simulink model "derivative_filter_test"  (R2023a)
settings: Solver=FixedStepDiscrete  StartTime=0.0  StopTime=1  FixedStep=T_s  RelTol=1e-3
InitFcn:
  | filter_init
values from neighbouring files (symbols this model uses):
  beta_v = T_s/(T_s+tau_v)    (= 0.5)    [filter_init.m]
  N_e = 12    [filter_init.m]
  T_s = 0.001    [filter_init.m]
  tau_der = 0.01    [filter_init.m]
undefined symbols (not defined in the file or in its folder): den_filt, den_filt_be, den_filt_fe, num_filt, num_filt_be, num_filt_fe
settings Model: Creator=mfocchi  LastModifiedBy=mfocchi

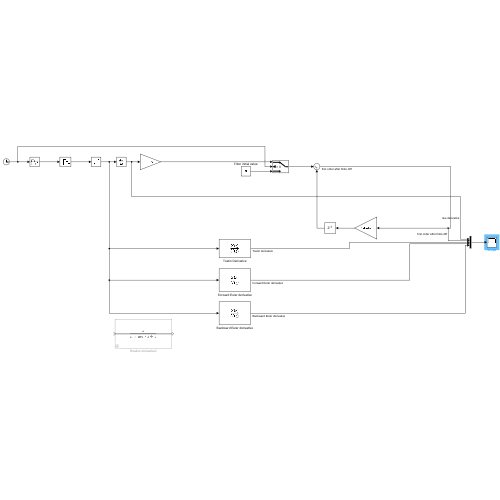
[thumbnail: Simulink's stored preview of the top-level diagram]
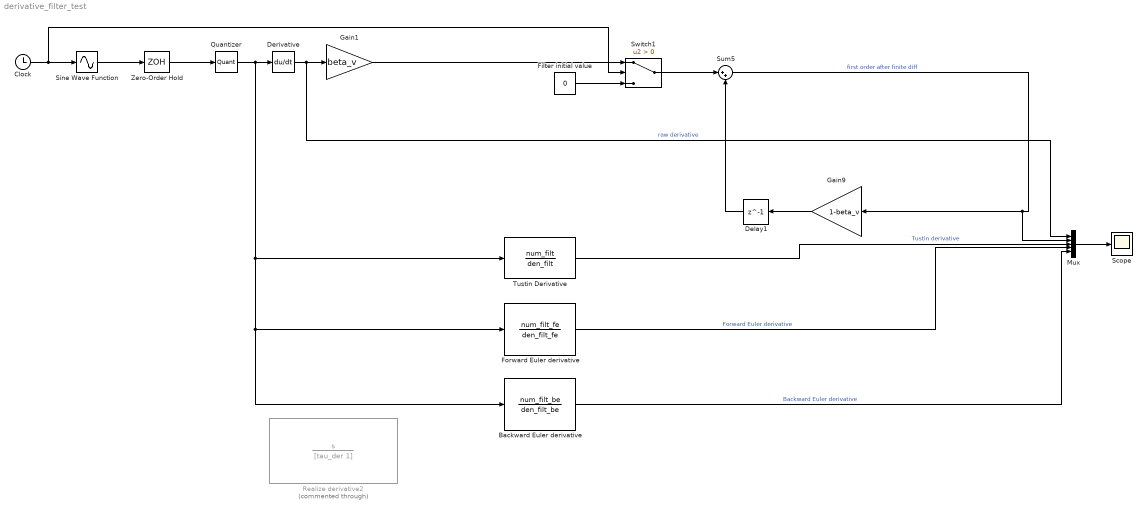
== system derivative_filter_test ==
  Backward Euler derivative : DiscreteTransferFcn  Numerator=num_filt_be  Denominator=den_filt_be  InitialStates=1  SampleTime=T_s
  Clock : Clock
  Delay1 : Delay  DelayLength=1  InitialCondition=0  SampleTime=T_s
  Derivative : Derivative
  Filter initial value : Constant  Value=0
  Forward Euler derivative : DiscreteTransferFcn  Numerator=num_filt_fe  Denominator=den_filt_fe  InitialStates=1  SampleTime=T_s
  Gain1 : Gain  Gain=beta_v
  Gain9 : Gain  Gain=1-beta_v
  Mux : Mux  Inputs=5
  Quantizer : Quantizer  QuantizationInterval=2*pi/(2^N_e)
  Realize derivative2 : TransferFcn  Commented=through  Numerator=[1 0]  Denominator=[tau_der 1]
  Scope : Scope
  Sine Wave Function : Sin  TimeSource=Use external signal  Frequency=2*pi  SampleTime=0
  Sum5 : Sum  Inputs=|++
  Switch1 : Switch  Criteria=u2 > Threshold  SaturateOnIntegerOverflow=off  InputSameDT=off
  Tustin Derivative : DiscreteTransferFcn  Numerator=num_filt  Denominator=den_filt  InitialStates=1  SampleTime=T_s
  Zero-Order Hold : ZeroOrderHold  SampleTime=T_s
  wires:
  Clock/1 -> Switch1/2, Sine Wave Function/1
  Sum5/1 -> Mux/2, Gain9/1  "first order after finite diff"
  Switch1/1 -> Sum5/1
  Delay1/1 -> Sum5/2
  Gain9/1 -> Delay1/1
  Filter initial value/1 -> Switch1/3
  Sine Wave Function/1 -> Zero-Order Hold/1
  Zero-Order Hold/1 -> Quantizer/1
  Derivative/1 -> Mux/1, Gain1/1  "raw derivative"
  Gain1/1 -> Switch1/1
  Mux/1 -> Scope/1
  Quantizer/1 -> Backward Euler derivative/1, Forward Euler derivative/1, Tustin Derivative/1, Derivative/1
  Tustin Derivative/1 -> Mux/3  "Tustin derivative"
  Forward Euler derivative/1 -> Mux/4  "Forward Euler derivative"
  Backward Euler derivative/1 -> Mux/5  "Backward Euler derivative"
